simulink model "helicopter_test_v4"  (Simulink 7.5)
settings: Solver=ode1  StartTime=0.0  StopTime=inf  FixedStep=0.1  RelTol=1e-3
undefined symbols (not defined in the file or in its folder): HIL
libraries: quarc_library x3
settings Model: Creator=ovidiua  LastModifiedBy=ovidiua  SimulationMode=external  ExtModeTrigDuration=5000
settings SolverCC: PositivePriorityOrder=on
settings RTWCC: SystemTargetFile=quarc_windows.tlc  TemplateMakefile=quarc_default_tmf  Description=QUARC Win32 Target  ProcessScript=quarc_windows_make_rtw_hook
settings STFCustomTargetCC: TargetPreCompLibLocation=C:\PROGRA~2\QUARC\lib\2010a\windows\release  GeneratePreprocessorConditionals=Disable all  SystemTargetFile=quarc_windows.tlc
settings GRTTargetCC: TargetPreCompLibLocation=C:\PROGRA~2\QUARC\lib\2010a\windows\release  ParMdlRefBuildCompliant=off  CompOptLevelCompliant=off  MatFileLogging=off  ExtMode=on  ExtModeMexFile=quarc_comm

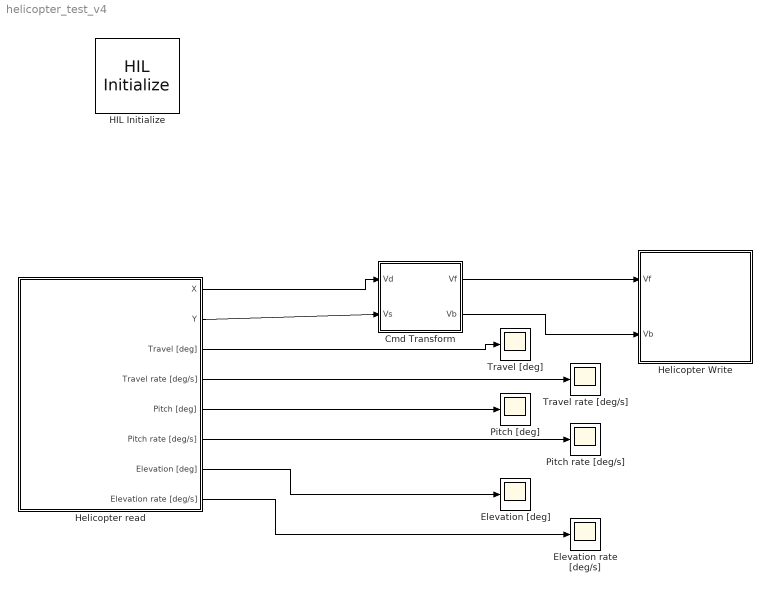
== system helicopter_test_v4 ==
  Cmd Transform : Subsystem
  Elevation [deg] : Scope
      settings: YMin=-30  YMax=7.5  SaveName=ScopeData2
  Elevation rate [deg/s] : Scope
      settings: YMin=-22.5  YMax=25  SaveName=ScopeData9
  HIL Initialize : quarc_library/Data Acquisition/Generic/Configuration/HIL Initialize  object_name=HIL-1  board_type=q4  board_number=0  exclusive=off  active=off  hardware_clocks=[0:1]  clock_modes=[0 0]  set_clock_params_at_start=on  set_clock_params_at_switch_in=off  analog_input_channels=[0:3]  analog_input_maximums=10  analog_input_minimums=-10  set_analog_input_params_at_start=off  set_analog_input_params_at_switch_in=off  analog_output_channels=[0:3]  analog_output_maximums=[10]  analog_output_minimums=[-10]  initial_analog_outputs=[0]  final_analog_outputs=[0]  watchdog_analog_outputs=0  set_analog_output_params_at_start=on  set_analog_output_params_at_switch_in=off  set_analog_outputs_at_start=on  set_analog_outputs_at_switch_in=off  set_analog_outputs_at_terminate=on  set_analog_outputs_at_switch_out=off  set_analog_outputs_on_watchdog=off  digital_input_channels=[]  digital_output_channels=[]  digital_output_configuration=[]  initial_digital_outputs=[1]  final_digital_outputs=[1]  watchdog_digital_outputs=[2]  set_digital_output_params_at_start=off  set_digital_output_params_at_switch_in=off  set_digital_outputs_at_start=on  set_digital_outputs_at_switch_in=off  set_digital_outputs_at_terminate=on  set_digital_outputs_at_switch_out=off  set_digital_outputs_on_watchdog=off  encoder_channels=[0:3]  quadrature=[4]  encoder_filter_frequency=(1/60e-9)/1  initial_encoder_counts=[0]  set_encoder_params_at_start=on  set_encoder_params_at_switch_in=off  set_encoder_counts_at_start=on  set_encoder_counts_at_switch_in=off  pwm_channels=[]  pwm_modes=[0]  pwm_frequency=(1/60e-9)/1024  pwm_configuration=[]  pwm_alignment=[]  pwm_polarity=[]  pwm_leading_deadband=[]  pwm_trailing_deadband=[]  initial_pwm_outputs=[0]  final_pwm_outputs=[0]  watchdog_pwm_outputs=[]  set_pwm_params_at_start=on  set_pwm_params_at_switch_in=off  set_pwm_outputs_at_start=on  set_pwm_outputs_at_switch_in=off  set_pwm_outputs_at_terminate=on  set_pwm_outputs_at_switch_out=off  set_pwm_outputs_on_watchdog=off  other_output_channels=[]  initial_other_outputs=[]  final_other_outputs=[]  watchdog_other_outputs=[]  set_other_outputs_at_start=off  set_other_outputs_at_switch_in=off  set_other_outputs_at_terminate=off  set_other_outputs_at_switch_out=off  set_other_outputs_on_watchdog=off
  Helicopter Write : Subsystem
  Helicopter read : Subsystem
  Pitch [deg] : Scope
      settings: YMin=-10  YMax=110  SaveName=ScopeData3
  Pitch rate [deg/s] : Scope
      settings: YMin=-90  YMax=50  SaveName=ScopeData8
  Travel [deg] : Scope
      settings: YMin=-14  YMax=3  SaveName=ScopeData4
  Travel rate [deg/s] : Scope
      settings: YMin=-30  YMax=35  SaveName=ScopeData7
  wires:
  Helicopter read/8(Elevation rate [deg/s]) -> Elevation rate [deg/s]/1
  Helicopter read/6(Pitch rate [deg/s]) -> Pitch rate [deg/s]/1
  Helicopter read/4(Travel rate [deg/s]) -> Travel rate [deg/s]/1
  Helicopter read/7(Elevation [deg]) -> Elevation [deg]/1
  Helicopter read/3(Travel [deg]) -> Travel [deg]/1
  Helicopter read/5(Pitch [deg]) -> Pitch [deg]/1
  Helicopter read/1(X) -> Cmd Transform/1(Vd)
  Helicopter read/2(Y) -> Cmd Transform/2(Vs)
  Cmd Transform/1(Vf) -> Helicopter Write/1("Vf ")
  Cmd Transform/2(Vb) -> Helicopter Write/2(Vb)

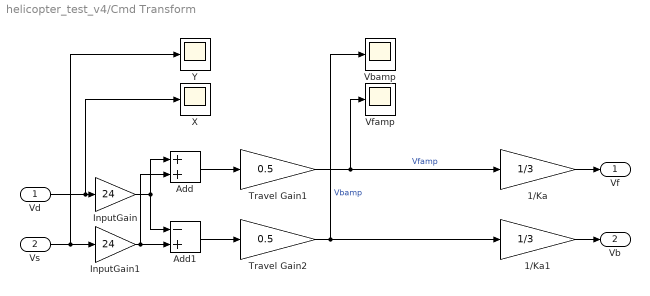
== system helicopter_test_v4/Cmd Transform ==
  Vd : Inport
  Vs : Inport  Port=2
  1/Ka : Gain  Gain=1/3  ParameterDataType=fixdt(1, 16)  ParameterScaling=2^0  OutDataType=fixdt(1, 16)  OutScaling=2^0
  1/Ka1 : Gain  Gain=1/3  ParameterDataType=fixdt(1, 16)  ParameterScaling=2^0  OutDataType=fixdt(1, 16)  OutScaling=2^0
  Add : Sum  OutDataType=fixdt(1, 16)  OutScaling=2^-10
  Add1 : Sum  Inputs=-+  OutDataType=fixdt(1, 16)  OutScaling=2^-10
  InputGain : Gain  Gain=24  ParameterDataType=fixdt(1, 16)  ParameterScaling=2^0  OutDataType=fixdt(1, 16)  OutScaling=2^0
  InputGain1 : Gain  Gain=24  ParameterDataType=fixdt(1, 16)  ParameterScaling=2^0  OutDataType=fixdt(1, 16)  OutScaling=2^0
  Travel Gain1 : Gain  Gain=0.5  ParameterDataType=fixdt(1, 16)  ParameterScaling=2^0  OutDataType=fixdt(1, 16)  OutScaling=2^0
  Travel Gain2 : Gain  Gain=0.5  ParameterDataType=fixdt(1, 16)  ParameterScaling=2^0  OutDataType=fixdt(1, 16)  OutScaling=2^0
  Vbamp : Scope
      settings: YMin=-1  YMax=12
  Vfamp : Scope
      settings: YMin=-1  YMax=12
  X : Scope
      settings: YMin=-0.1  YMax=1.1  SaveName=ScopeData5
  Y : Scope
      settings: YMin=-0.035  YMax=-0.005  SaveName=ScopeData6
  Vf : Outport
  Vb : Outport  Port=2
  wires:
  Add/1 -> Travel Gain1/1
  Add1/1 -> Travel Gain2/1
  Travel Gain1/1 -> 1/Ka/1, Vfamp/1  "Vfamp"
  Travel Gain2/1 -> 1/Ka1/1, Vbamp/1  "Vbamp"
  Vd/1 -> X/1, InputGain/1
  Vs/1 -> Y/1, InputGain1/1
  InputGain/1 -> Add/1, Add1/1
  InputGain1/1 -> Add1/2, Add/2
  1/Ka/1 -> Vf/1
  1/Ka1/1 -> Vb/1

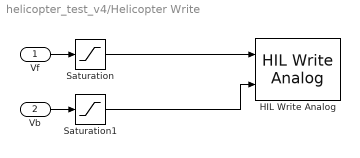
== system helicopter_test_v4/Helicopter Write ==
  "Vf " : Inport
  Vb : Inport  Port=2
  HIL Write Analog : quarc_library/Data Acquisition/Generic/Immediate I//O/HIL Write Analog  object_name=HIL-1  channels=[0,1]  sample_time=-1  active=off  vector_input=off
  Saturation : Saturate  UpperLimit=3  LowerLimit=-3  OutDataType=fixdt(1, 16)  OutScaling=2^0
  Saturation1 : Saturate  UpperLimit=3  LowerLimit=-3  OutDataType=fixdt(1, 16)  OutScaling=2^0
  wires:
  Saturation/1 -> HIL Write Analog/1
  Saturation1/1 -> HIL Write Analog/2
  "Vf "/1 -> Saturation/1
  Vb/1 -> Saturation1/1

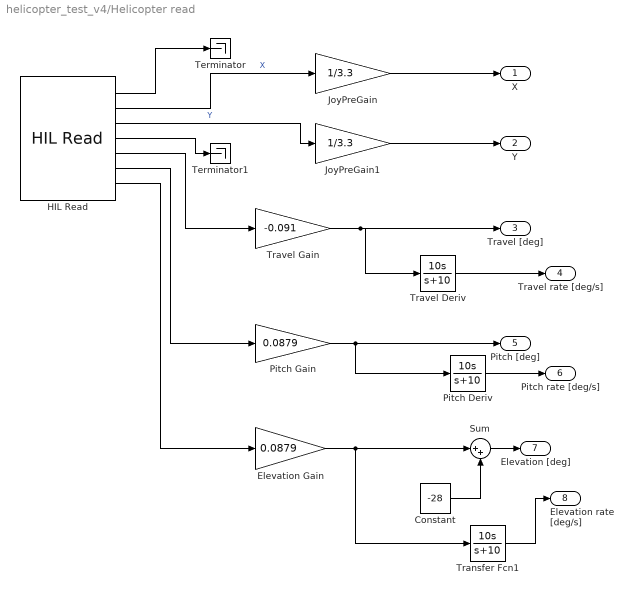
== system helicopter_test_v4/Helicopter read ==
  Constant : Constant  Value=-28  OutDataType=fixdt(1, 16)  OutScaling=2^0
  Elevation Gain : Gain  Gain=0.0879  ParameterDataType=fixdt(1, 16)  ParameterScaling=2^0  OutDataType=fixdt(1, 16)  OutScaling=2^0
  HIL Read : quarc_library/Data Acquisition/Generic/Immediate I//O/HIL Read  object_name=HIL-1  analog_channels=[0:3]  encoder_channels=[0:2]  digital_channels=[]  other_channels=[]  sample_time=qc_get_step_size  active=on  vector_output=off  data_type_mode=Inherit via back propagation  encoder_data_type=double  digital_data_type=boolean
  JoyPreGain : Gain  Gain=1/3.3  ParameterDataType=fixdt(1, 16)  ParameterScaling=2^0  OutDataType=fixdt(1, 16)  OutScaling=2^0
  JoyPreGain1 : Gain  Gain=1/3.3  ParameterDataType=fixdt(1, 16)  ParameterScaling=2^0  OutDataType=fixdt(1, 16)  OutScaling=2^0
  Pitch Deriv : TransferFcn  Numerator=[10 0]  Denominator=[1 10]
  Pitch Gain : Gain  Gain=0.0879  ParameterDataType=fixdt(1, 16)  ParameterScaling=2^0  OutDataType=fixdt(1, 16)  OutScaling=2^0
  Sum : Sum  Inputs=|++  OutDataType=fixdt(1, 16)  OutScaling=2^0
  Terminator : Terminator
  Terminator1 : Terminator
  Transfer Fcn1 : TransferFcn  Numerator=[10 0]  Denominator=[1 10]
  Travel Deriv : TransferFcn  Numerator=[10 0]  Denominator=[1 10]
  Travel Gain : Gain  Gain=-0.091  ParameterDataType=fixdt(1, 16)  ParameterScaling=2^0  OutDataType=fixdt(1, 16)  OutScaling=2^0
  X : Outport
  Y : Outport  Port=2
  Travel [deg] : Outport  Port=3
  Travel rate [deg/s] : Outport  Port=4
  Pitch [deg] : Outport  Port=5
  Pitch rate [deg/s] : Outport  Port=6
  Elevation [deg] : Outport  Port=7
  Elevation rate [deg/s] : Outport  Port=8
  wires:
  HIL Read/1 -> Terminator/1
  HIL Read/4 -> Terminator1/1
  HIL Read/5 -> Travel Gain/1
  HIL Read/6 -> Pitch Gain/1
  HIL Read/7 -> Elevation Gain/1
  Travel Gain/1 -> Travel Deriv/1, Travel [deg]/1
  Elevation Gain/1 -> Transfer Fcn1/1, Sum/1
  Pitch Gain/1 -> Pitch Deriv/1, Pitch [deg]/1
  Constant/1 -> Sum/2
  Travel Deriv/1 -> Travel rate [deg/s]/1
  Pitch Deriv/1 -> Pitch rate [deg/s]/1
  Sum/1 -> Elevation [deg]/1
  Transfer Fcn1/1 -> Elevation rate [deg/s]/1
  HIL Read/2 -> JoyPreGain/1  "X"
  HIL Read/3 -> JoyPreGain1/1  "Y"
  JoyPreGain1/1 -> Y/1
  JoyPreGain/1 -> X/1
